simulink model "vision_test"  (Simulink 7.6)
settings: Solver=FixedStepDiscrete  StartTime=0.0  StopTime=0  RelTol=1e-3
undefined symbols (not defined in the file or in its folder): gray, jet, Rec, SDTV
libraries: vipsnks x6, vipconversions x2, vipsrcs x2
settings Model: Creator=Administrator  LastModifiedBy=auvt

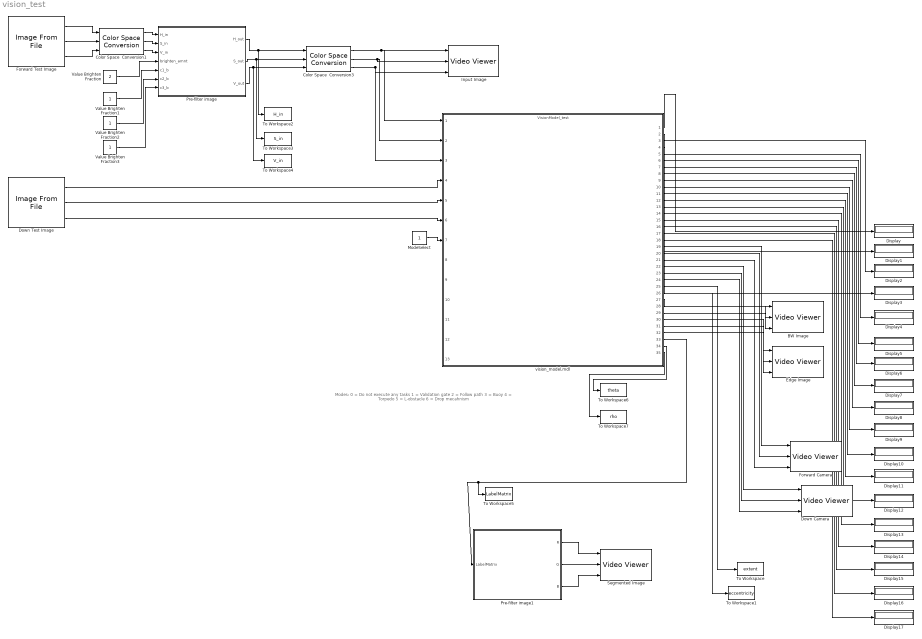
== system vision_test ==
  note: Modes:
      | 0 = Do not execute any tasks
      | 1 = Validation gate
      | 2 = Follow path
      | 3 = Buoy
      | 4 = Torpedo
      | 5 = L-obstacle
      | 6 = Drop mecahnism
  BW Image : vipsnks/Video Viewer  DialogControllerArgs=DataTag1  inputType=Obsolete7b  imagePorts=Separate color signals  useColorMap=off  colormapValue=gray(256)  specRange=off  minInputVal=0  maxInputVal=255  FigPos=[613 318 262 182]  AxisZoom=on  trueSizedOnce=off  OpenAtMdlStart=on
  Color Space  Conversion1 : vipconversions/Color Space  Conversion  conversion=Obsolete  conversionActive=R'G'B' to HSV  wp_str=D50  rec=Rec. 601 (SDTV)  sys=1125/60/2:1  imagePorts=Separate color signals
  Color Space  Conversion3 : vipconversions/Color Space  Conversion  conversion=Obsolete  conversionActive=HSV to R'G'B'  wp_str=D50  rec=Rec. 601 (SDTV)  sys=1125/60/2:1  imagePorts=Separate color signals
  Display{,1..17} (18 alike) : Display
  Down Camera : vipsnks/Video Viewer  DialogControllerArgs=DataTag3  inputType=Obsolete7b  imagePorts=Separate color signals  useColorMap=off  colormapValue=jet(256)  specRange=off  minInputVal=0  maxInputVal=255  FigPos=[33 609 253 188]  AxisZoom=on  trueSizedOnce=off  OpenAtMdlStart=on
  Down Test Image : vipsrcs/Image From File  Tag=vipblks_nd  DialogController=vipDDGCreate  DialogControllerArgs=DataTag4  SystemSampleTime=-1  FileName=/home/auvt/auvc/src/vision/Modified_Files_for_Testing/Images/gate1.PNG  imagePorts=Separate color signals  Ts=-1  ImageDataType=double  Signed=on  WordLength=16  sdImageDataType=uint(8)  FractionLengthMode=User-defined  FractionLength=15  OutPortLabels=R|G|B
  Edge Image : vipsnks/Video Viewer  DialogControllerArgs=DataTag6  inputType=Obsolete7b  imagePorts=Separate color signals  useColorMap=off  colormapValue=gray(256)  specRange=off  minInputVal=0  maxInputVal=255  FigPos=[899 318 262 182]  AxisZoom=on  trueSizedOnce=off  OpenAtMdlStart=on
  Forward Camera : vipsnks/Video Viewer  DialogControllerArgs=DataTag8  inputType=Obsolete7b  imagePorts=Separate color signals  useColorMap=off  colormapValue=gray(256)  specRange=off  minInputVal=0  maxInputVal=255  FigPos=[326 318 262 182]  AxisZoom=on  trueSizedOnce=off  OpenAtMdlStart=on
  Forward Test Image : vipsrcs/Image From File  Tag=vipblks_nd  DialogController=vipDDGCreate  DialogControllerArgs=DataTag9  SystemSampleTime=-1  FileName=/home/auvt/auvc/src/vision/Modified_Files_for_Testing/Images/gate9.PNG  imagePorts=Separate color signals  Ts=-1  ImageDataType=double  Signed=on  WordLength=16  sdImageDataType=uint(8)  FractionLengthMode=User-defined  FractionLength=15  OutPortLabels=R|G|B
  Input Image : vipsnks/Video Viewer  DialogControllerArgs=DataTag11  inputType=Obsolete7b  imagePorts=Separate color signals  useColorMap=off  colormapValue=jet(256)  specRange=off  minInputVal=0  maxInputVal=255  FigPos=[23 307 275 171]  AxisZoom=on  trueSizedOnce=off  OpenAtMdlStart=on
  ModeSelect : Constant  SampleTime=-1
  Pre-filter image : Stateflow chart  TreatAsAtomicUnit=on
  Pre-filter image1 : Stateflow chart  TreatAsAtomicUnit=on
  Segmented Image : vipsnks/Video Viewer  DialogControllerArgs=DataTag13  inputType=Obsolete7b  imagePorts=Separate color signals  useColorMap=off  colormapValue=jet(256)  specRange=off  minInputVal=0  maxInputVal=255  FigPos=[317 631 301 208]  AxisZoom=on  trueSizedOnce=off  OpenAtMdlStart=on
  To Workspace : ToWorkspace  VariableName=extent  SampleTime=-1  SaveFormat=Array
  To Workspace1 : ToWorkspace  VariableName=eccentricity  SampleTime=-1  SaveFormat=Array
  To Workspace2 : ToWorkspace  VariableName=H_in  SampleTime=-1  SaveFormat=Array
  To Workspace3 : ToWorkspace  VariableName=S_in  SampleTime=-1  SaveFormat=Array
  To Workspace4 : ToWorkspace  VariableName=V_in  SampleTime=-1  SaveFormat=Array
  To Workspace5 : ToWorkspace  VariableName=LabelMatrix  SampleTime=-1  SaveFormat=Array
  To Workspace6 : ToWorkspace  VariableName=theta  SampleTime=-1  SaveFormat=Array
  To Workspace7 : ToWorkspace  VariableName=rho  SampleTime=-1  SaveFormat=Array
  Value Brighten Fraction : Constant  Value=2  SampleTime=-1
  Value Brighten Fraction1 : Constant  SampleTime=-1
  Value Brighten Fraction2 : Constant  SampleTime=-1
  Value Brighten Fraction3 : Constant  SampleTime=-1
  vision_model.mdl : ModelReference  ModelNameDialog=VisionModel_test  SimulationMode=Accelerator  ModelReferenceVersion=1.360  CopyOfModelName=VisionModel_test
  wires:
  ModeSelect/1 -> vision_model.mdl/7
  vision_model.mdl/1 -> Display/1
  vision_model.mdl/2 -> Display1/1
  vision_model.mdl/3 -> Display2/1
  vision_model.mdl/4 -> Display3/1
  vision_model.mdl/5 -> Display4/1
  vision_model.mdl/6 -> Display5/1
  vision_model.mdl/7 -> Display6/1
  vision_model.mdl/8 -> Display7/1
  vision_model.mdl/9 -> Display8/1
  vision_model.mdl/10 -> Display9/1
  vision_model.mdl/11 -> Display10/1
  vision_model.mdl/12 -> Display11/1
  vision_model.mdl/13 -> Display12/1
  vision_model.mdl/14 -> Display13/1
  vision_model.mdl/15 -> Display14/1
  vision_model.mdl/16 -> Display15/1
  vision_model.mdl/17 -> Display16/1
  vision_model.mdl/18 -> Display17/1
  Down Test Image/1 -> vision_model.mdl/4
  Down Test Image/2 -> vision_model.mdl/5
  Down Test Image/3 -> vision_model.mdl/6
  vision_model.mdl/19 -> Forward Camera/1
  vision_model.mdl/20 -> Forward Camera/2
  vision_model.mdl/21 -> Forward Camera/3
  vision_model.mdl/22 -> Down Camera/1
  vision_model.mdl/23 -> Down Camera/2
  vision_model.mdl/24 -> Down Camera/3
  vision_model.mdl/25 -> To Workspace/1
  vision_model.mdl/26 -> To Workspace1/1
  Value Brighten Fraction/1 -> Pre-filter image/4(brighten_amnt)
  Value Brighten Fraction1/1 -> Pre-filter image/5(c1_b)
  Value Brighten Fraction2/1 -> Pre-filter image/6(c2_b)
  Value Brighten Fraction3/1 -> Pre-filter image/7(c3_b)
  Forward Test Image/2 -> Color Space  Conversion1/2
  Forward Test Image/1 -> Color Space  Conversion1/1
  Forward Test Image/3 -> Color Space  Conversion1/3
  Color Space  Conversion1/3 -> Pre-filter image/3(V_in)
  Color Space  Conversion1/2 -> Pre-filter image/2(S_in)
  Color Space  Conversion1/1 -> Pre-filter image/1(H_in)
  Pre-filter image/1(H_out) -> Color Space  Conversion3/1, To Workspace2/1
  Pre-filter image/2(S_out) -> Color Space  Conversion3/2, To Workspace3/1
  Pre-filter image/3(V_out) -> Color Space  Conversion3/3, To Workspace4/1
  Color Space  Conversion3/1 -> vision_model.mdl/1, Input Image/1
  Color Space  Conversion3/2 -> vision_model.mdl/2, Input Image/2
  Color Space  Conversion3/3 -> vision_model.mdl/3, Input Image/3
  vision_model.mdl/27 -> BW Image/1
  vision_model.mdl/28 -> BW Image/2
  vision_model.mdl/29 -> BW Image/3
  vision_model.mdl/30 -> Edge Image/1
  vision_model.mdl/31 -> Edge Image/2
  vision_model.mdl/32 -> Edge Image/3
  Pre-filter image1/1(R) -> Segmented Image/1
  Pre-filter image1/2(G) -> Segmented Image/2
  Pre-filter image1/3(B) -> Segmented Image/3
  vision_model.mdl/33 -> To Workspace5/1, Pre-filter image1/1(LabelMatrix)
  vision_model.mdl/34 -> To Workspace6/1
  vision_model.mdl/35 -> To Workspace7/1

== matlab function Pre-filter image ==
  data: H_in input double; S_in input double; V_in input double; H_out output double; S_out output double; V_out output double; brighten_amnt input double; c1_b input double; c2_b input double; c3_b input double
function [H_out, S_out, V_out] = brightenImage(H_in, S_in, V_in, brighten_amnt, c1_b, c2_b, c3_b)
%#eml

%H_out = c1_b.*H_in;
%S_out = c2_b.*S_in;
%V_out = c3_b.*V_in;



H_out = H_in;
S_out = S_in;
V_out = brighten_amnt.*V_in;




return

== matlab function Pre-filter image1 ==
  data: LabelMatrix input double; R output double; G output double; B output double
function [R, G, B] = display_LabelMatrix(LabelMatrix)
%#eml



R = LabelMatrix./max(max(max(abs(LabelMatrix))));
G = R;
B = R;



return
